simulink model "SILS_201704211"  (R2022b)
settings: Solver=ode4  StartTime=0.0  StopTime=10000  FixedStep=sim_dt  RelTol=1e-3  EnableMultiTasking=on
PreLoadFcn:
  | start
  | make_SILS
  | param_SW
  | param_sys
  | param_component
  | param_env
  | param_alignment
  | OEread
  | initialCondition
undefined symbols (not defined in the file or in its folder): ADSW, AOBC_dt, area, GAS_b2c, GGSW, GPperturbationSW, GYRO_b2c, MTQ_c2b, noise_sampling_rate, NSAS1_b2c, NSAS2_b2c, NSAS3_b2c, NSAS4_b2c, NSAS5_b2c, NSAS6_b2c, rem_mag, rem_magSW, RW_J, SRPSW, STT1_b2c_quat, STT_seed1, STT_x_noise, STT_y_noise, STT_z_noise
libraries: lib_util x23, lib_component x14, lib_env x9, aerolibutil x4, lib_orbittrance x3, aerolibtransform2 x1, sharedtransform x1
CloseFcn:
  | clean
settings Model: Creator=yamaurashusaku  LastModifiedBy=hapham
settings SolverCC: AlgebraicLoopSolver=TrustRegion
settings DataIOCC: LimitDataPoints=on  SaveFinalState=on  SaveFormat=Array  SignalLoggingSaveFormat=ModelDataLogs  SaveState=on  ReturnWorkspaceOutputs=off  StateSaveName=tmp_raccel_xout
settings OptimizationCC: ExpressionDepthLimit=2147483647  EfficientMapNaN2IntZero=off  LifeSpan=inf
settings DebuggingCC: UnderspecifiedInitializationDetection=Classic  MergeDetectMultiDrivingBlocksExec=none  SolverPrmCheckMsg=warning  MultiTaskCondExecSysMsg=warning  FcnCallInpInsideContextMsg=warning  UnconnectedInputMsg=warning  UnconnectedOutputMsg=warning  UnconnectedLineMsg=warning  StateNameClashWarn=warning  SFUnexpectedBacktrackingDiag=warning  SFNoUnconditionalDefaultTransitionDiag=warning  SFExecutionAtInitializationDiag=none  SFMachineParentedDataDiag=warning  ArithmeticOperatorsInVariantConditions=warning
settings HardwareCC: ProdBitPerPointer=32  ProdBitPerSizeT=32  ProdBitPerPtrDiffT=32  ProdLargestAtomicFloat=None  ProdIntDivRoundTo=Undefined  ProdEndianess=Unspecified  ProdWordSize=32  ProdHWDeviceType=32-bit Generic  TargetBitPerPointer=64  TargetBitPerSizeT=64  TargetBitPerPtrDiffT=64  TargetLongLongMode=on  TargetIntDivRoundTo=Zero  TargetEndianess=LittleEndian  TargetWordSize=64  TargetHWDeviceType=MATLAB Host  ProdEqTarget=off
settings ModelReferenceCC: EnableRefExpFcnMdlSchedulingChecks=on  PropagateSignalLabelsOutOfModel=off
settings SFSimCC: SimUseLocalCustomCode=off  CustomCodeUndefinedFunction=UseInterfaceOnly
settings SFSimCC: SimUserSources=|
  | sfunc_nrlmsise00_wrapper.c
  | nrlmsise-00.c
  | nrlmsise-00_data.c
  | createHandle.c
  | globals.c
  | AOCS_Process.c
settings RTWCC: SystemTargetFile=raccel.tlc  RTWVerbose=off  RTWUseLocalCustomCode=off  RTWUseSimCustomCode=on  DLArmComputeVersion=19.05
settings RTWCC: CustomSource=|
  | sfunc_nrlmsise00_wrapper.c
  | nrlmsise-00.c
  | nrlmsise-00_data.c
  | createHandle.c
  | globals.c
  | AOCS_Process.c
settings CodeAppCC: GenerateComments=off  MaxIdLength=128  SimulinkBlockComments=off
settings RaccelTargetCC: ParMdlRefBuildCompliant=off  LogVarNameModifier=rt_  OptimizeReductions=off  ENABLE_SLEXEC_SSBRIDGE=0  RTWCAPISignals=off  RTWCAPIParams=off  RTWCAPIRootIO=off
settings ConfigComp: CovMetricSettings=dw  CovSaveCumulativeToWorkspaceVar=on  CovSaveSingleToWorkspaceVar=on  CovExternalEMLEnable=off

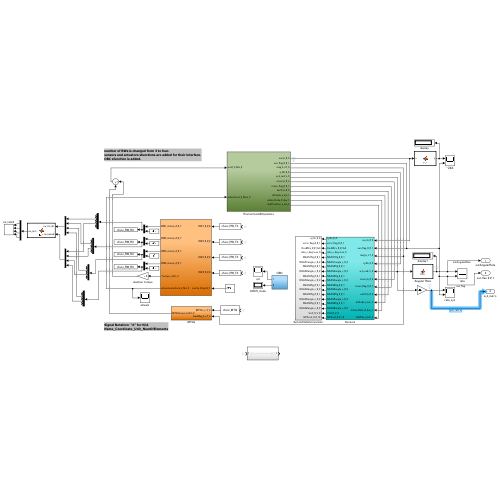
[thumbnail: Simulink's stored preview of the top-level diagram]
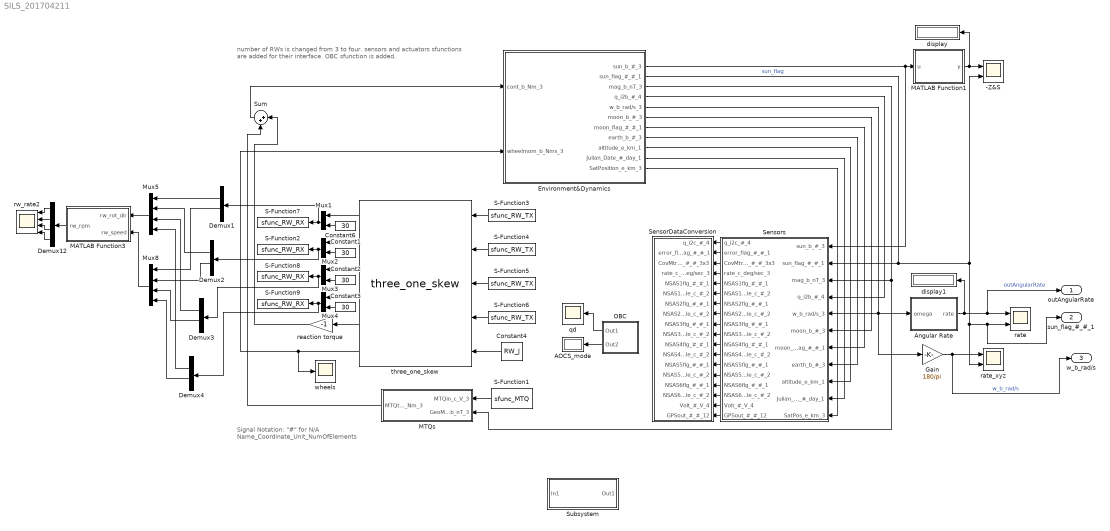
== system SILS_201704211 ==
  note: Signal Notation: "#" for N/A
      | Name_Coordinate_Unit_NumOfElements
  note: number of RWs is changed from 3 to four.
      | sensors and actuators sfunctions are added for their interface.
      | OBC sfunction is added.
  -Z&S : Scope  NumInputPorts=2
  AOCS_mode : Display
  Angular Rate : MATLAB Function  TreatAsAtomicUnit=on
  Constant{1..3,6} (4 alike) : Constant  Value=30
  Constant4 : Constant  Value=RW_J
  Demux{1..4} (4 alike) : Demux  Outputs=8
  Demux12 : Demux
  Environment&Dynamics : Subsystem
  Gain : Gain  Gain=180/pi
  MATLAB Function1 : MATLAB Function  TreatAsAtomicUnit=on
  MATLAB Function3 : MATLAB Function  TreatAsAtomicUnit=on
  MTQs : Subsystem
  Mux{1..4} (4 alike) : Mux  Inputs=2
  Mux5 : Mux
  Mux8 : Mux
  OBC : Subsystem
  S-Function1 : S-Function  FunctionName=sfunc_MTQ  Parameters=0  SFunctionDeploymentMode=off  EnableBusSupport=off
  S-Function2 : S-Function  FunctionName=sfunc_RW_RX  Parameters=1  SFunctionDeploymentMode=off  EnableBusSupport=off
  S-Function3 : S-Function  FunctionName=sfunc_RW_TX  Parameters=0  SFunctionDeploymentMode=off  EnableBusSupport=off
  S-Function4 : S-Function  FunctionName=sfunc_RW_TX  Parameters=1  SFunctionDeploymentMode=off  EnableBusSupport=off
  S-Function5 : S-Function  FunctionName=sfunc_RW_TX  Parameters=2  SFunctionDeploymentMode=off  EnableBusSupport=off
  S-Function6 : S-Function  FunctionName=sfunc_RW_TX  Parameters=3  SFunctionDeploymentMode=off  EnableBusSupport=off
  S-Function7 : S-Function  FunctionName=sfunc_RW_RX  Parameters=0  SFunctionDeploymentMode=off  EnableBusSupport=off
  S-Function8 : S-Function  FunctionName=sfunc_RW_RX  Parameters=2  SFunctionDeploymentMode=off  EnableBusSupport=off
  S-Function9 : S-Function  FunctionName=sfunc_RW_RX  Parameters=3  SFunctionDeploymentMode=off  EnableBusSupport=off
  SensorDataConversion : Subsystem
  Sensors : Subsystem
  Subsystem : Subsystem
  Sum : Sum  Inputs=|++
  display : Display
  display1 : Display
  qd : Scope
  rate : Scope  NumInputPorts=2
  rate_xyz : Scope  NumInputPorts=2
  reaction torque : Gain  Gain=-1
  rw_rate2 : Scope  NumInputPorts=4
  three_one_skew : lib_component/three_one_skew  SystemSampleTime=-1  VariantActivationTime=update diagram  Latency=0  AutoFrameSizeCalculation=off
  wheels : Scope
  outAngularRate : Outport
  sun_flag_#_#_1 : Outport  Port=2
  w_b_rad/s : Outport  Port=3
  wires:
  three_one_skew/6 -> Environment&Dynamics/2(wheelmom_b_Nms_3), wheels/1
  Environment&Dynamics/1(sun_b_#_3) -> Sensors/1(sun_b_#_3), MATLAB Function1/1(u)
  Environment&Dynamics/2(sun_flag_#_#_1) -> -Z&S/2, sun_flag_#_#_1/1, rate/2, rate_xyz/2, Sensors/2(sun_flag_#_#_1)  "sun_flag"
  Environment&Dynamics/3(mag_b_nT_3) -> Sensors/3(mag_b_nT_3), MTQs/2(GeoMag_b_nT_3)
  Environment&Dynamics/4(q_i2b_#_4) -> Sensors/4(q_i2b_#_4)
  Environment&Dynamics/5(w_b_rad/s_3) -> Angular Rate/1(omega), Sensors/5(w_b_rad/s_3), Gain/1
  Environment&Dynamics/6(moon_b_#_3) -> Sensors/6(moon_b_#_3)
  Environment&Dynamics/7(moon_flag_#_#_1) -> Sensors/7(moon_flag_#_#_1)
  Environment&Dynamics/8(earth_b_#_3) -> Sensors/8(earth_b_#_3)
  Environment&Dynamics/9(altitude_e_km_1) -> Sensors/9(altitude_e_km_1)
  Environment&Dynamics/10(Julian_Date_#_day_1) -> Sensors/10(Julian_Date_#_day_1)
  Environment&Dynamics/11(SatPosition_e_km_3) -> Sensors/11(SatPos_e_km_3)
  three_one_skew/5 -> reaction torque/1
  MTQs/1(MTQtorque_b_Nm_3) -> Sum/2
  Sum/1 -> Environment&Dynamics/1(cont_b_Nm_3)
  OBC/1(Out1) -> qd/1
  S-Function1/1 -> MTQs/1(MTQin_c_V_3)
  S-Function3/1 -> three_one_skew/1
  S-Function4/1 -> three_one_skew/2
  S-Function5/1 -> three_one_skew/3
  S-Function6/1 -> three_one_skew/4
  Mux1/1 -> Demux1/1, S-Function7/1
  three_one_skew/1 -> Mux1/1
  Constant6/1 -> Mux1/2
  Mux2/1 -> Demux2/1, S-Function2/1
  three_one_skew/2 -> Mux2/1
  Constant1/1 -> Mux2/2
  Mux3/1 -> Demux3/1, S-Function8/1
  three_one_skew/3 -> Mux3/1
  Constant2/1 -> Mux3/2
  Mux4/1 -> Demux4/1, S-Function9/1
  three_one_skew/4 -> Mux4/1
  Constant3/1 -> Mux4/2
  Constant4/1 -> three_one_skew/5
  reaction torque/1 -> Sum/1
  Gain/1 -> w_b_rad/s/1, rate_xyz/1  "w_b_rad/s"
  OBC/2(Out2) -> AOCS_mode/1
  Sensors/1(q_i2c_#_4) -> SensorDataConversion/1(q_i2c_#_4)
  Sensors/2(error_flag_#_#_1) -> SensorDataConversion/2(error_flag_#_#_1)
  Sensors/3(CovMtrx_#_#_3x3) -> SensorDataConversion/3(CovMtrx_#_#_3x3)
  Sensors/4(rate_c_deg/sec_3) -> SensorDataConversion/4(rate_c_deg/sec_3)
  Sensors/5(NSAS1flg_#_#_1) -> SensorDataConversion/5(NSAS1flg_#_#_1)
  Sensors/6(NSAS1angle_c_#_2) -> SensorDataConversion/6(NSAS1angle_c_#_2)
  Sensors/7(NSAS2flg_#_#_1) -> SensorDataConversion/7(NSAS2flg_#_#_1)
  Sensors/8(NSAS2angle_c_#_2) -> SensorDataConversion/8(NSAS2angle_c_#_2)
  Sensors/9(NSAS3flg_#_#_1) -> SensorDataConversion/9(NSAS3flg_#_#_1)
  Sensors/10(NSAS3angle_c_#_2) -> SensorDataConversion/10(NSAS3angle_c_#_2)
  Sensors/11(NSAS4flg_#_#_1) -> SensorDataConversion/11(NSAS4flg_#_#_1)
  Sensors/12(NSAS4angle_c_#_2) -> SensorDataConversion/12(NSAS4angle_c_#_2)
  Sensors/13(NSAS5flg_#_#_1) -> SensorDataConversion/13(NSAS5flg_#_#_1)
  Sensors/14(NSAS5angle_c_#_2) -> SensorDataConversion/14(NSAS5angle_c_#_2)
  Sensors/15(NSAS6flg_#_#_1) -> SensorDataConversion/15(NSAS6flg_#_#_1)
  Sensors/16(NSAS6angle_c_#_2) -> SensorDataConversion/16(NSAS6angle_c_#_2)
  Sensors/17(Volt_#_V_4) -> SensorDataConversion/17(Volt_#_V_4)
  Sensors/18(GPSout_#_#_12) -> SensorDataConversion/18(GPSout_#_#_12)
  Angular Rate/1(rate) -> display1/1, outAngularRate/1, rate/1  "outAngularRate"
  Demux1/3 -> Mux5/1
  Demux3/3 -> Mux5/3
  Demux4/3 -> Mux5/4
  Demux1/6 -> Mux8/1
  Demux2/6 -> Mux8/2
  Demux3/6 -> Mux8/3
  Demux4/6 -> Mux8/4
  MATLAB Function3/1(rw_rpm) -> Demux12/1
  Demux12/1 -> rw_rate2/1
  Demux12/2 -> rw_rate2/2
  Demux12/3 -> rw_rate2/3
  Demux12/4 -> rw_rate2/4
  Mux5/1 -> MATLAB Function3/1(rw_rot_dir)
  Mux8/1 -> MATLAB Function3/2(rw_speed)
  Demux2/3 -> Mux5/2
  MATLAB Function1/1(y) -> display/1, -Z&S/1

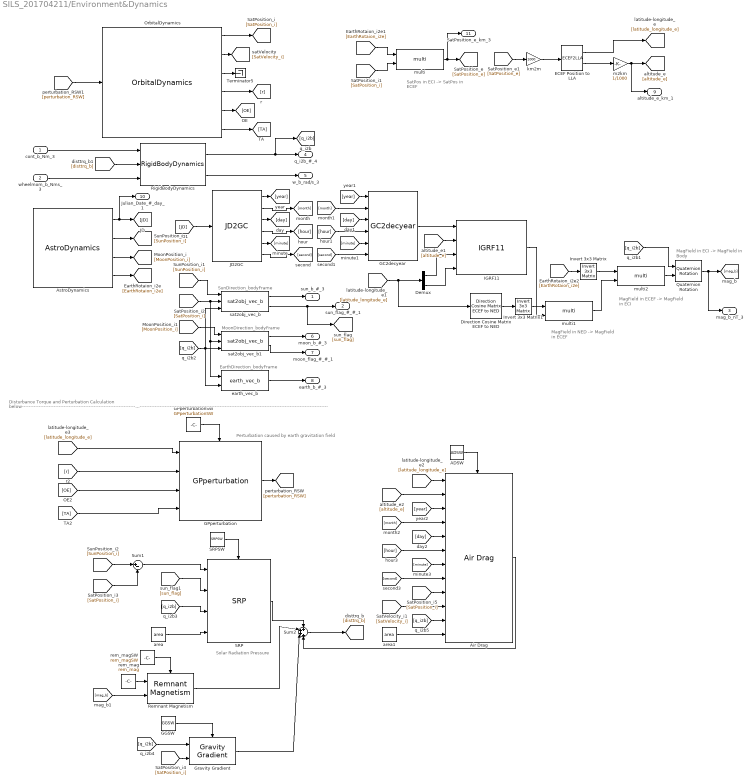
== system SILS_201704211/Environment&Dynamics ==
  note: MagField in ECI ->
      | MagField in Body
  note: MagField in ECEF ->
      | MagField in ECI
  note: MagField in NED ->
      | MagField in ECEF
  note: SatPos in ECI ->
      | SatPos in ECEF
  note: EarthDirection_bodyFrame
  note: MoonDirection_bodyFrame
  note: SunDirection_bodyFrame
  note: Disturbance Torque and Perturbation Calculation below-------------------------------------------------------------------------------------------------------------------------------------------------------------------------------------------------------------------------------------------------------------------------------------------------------------------------------------------------------
  note: Perturbation caused by earth gravitation field
  note: Solar Radiation Pressure
  cont_b_Nm_3 : Inport
  wheelmom_b_Nms_3 : Inport  Port=2
  ADSW : Constant  Value=ADSW
  Air Drag : lib_env/Environment&Dynamics/Air Drag  SystemSampleTime=-1  VariantActivationTime=update diagram  Latency=0  AutoFrameSizeCalculation=off
  AstroDynamics : lib_env/Environment&Dynamics/AstroDynamics  SystemSampleTime=-1  VariantActivationTime=update diagram  Latency=0  AutoFrameSizeCalculation=off
  Demux : Demux  Outputs=2
  Direction Cosine Matrix ECEF to NED : aerolibtransform2/Direction Cosine Matrix ECEF to NED
  ECEF Position to LLA : ECEF2LLA  R=6378137
  GC2decyear : lib_util/GC2decyear  SystemSampleTime=-1  VariantActivationTime=update diagram  Latency=0  AutoFrameSizeCalculation=off
  GGSW : Constant  Value=GGSW
  GPperturbation : lib_env/Environment&Dynamics/GPperturbation  SystemSampleTime=-1  VariantActivationTime=update diagram  Latency=0  AutoFrameSizeCalculation=off
  GPperturbationSW : Constant  Value=GPperturbationSW
  Gravity Gradient : lib_env/Environment&Dynamics/Gravity Gradient  SystemSampleTime=-1  VariantActivationTime=update diagram  Latency=0  AutoFrameSizeCalculation=off
  IGRF11 : lib_env/IGRF11  SystemSampleTime=-1  VariantActivationTime=update diagram  Latency=0  AutoFrameSizeCalculation=off
  Invert 3x3 Matrix : aerolibutil/Invert  3x3 Matrix
  Invert 3x3 Matrix1 : aerolibutil/Invert  3x3 Matrix
  JD2GC : lib_util/JD2GC  SystemSampleTime=-1  VariantActivationTime=update diagram  Latency=0  AutoFrameSizeCalculation=off
  OrbitalDynamics : lib_env/Environment&Dynamics/OrbitalDynamics  SystemSampleTime=-1  VariantActivationTime=update diagram  Latency=0  AutoFrameSizeCalculation=off
  Quaternion Rotation : aerolibutil/Quaternion Rotation
  Remnant Magnetism : lib_env/Environment&Dynamics/Remnant Magnetism  SystemSampleTime=-1  VariantActivationTime=update diagram  Latency=0  AutoFrameSizeCalculation=off
  RigidBodyDynamics : lib_env/Environment&Dynamics/RigidBodyDynamics  SystemSampleTime=-1  VariantActivationTime=update diagram  Latency=0  AutoFrameSizeCalculation=off
  SRP : lib_env/Environment&Dynamics/SRP  SystemSampleTime=-1  VariantActivationTime=update diagram  Latency=0  AutoFrameSizeCalculation=off
  SRPSW : Constant  Value=SRPSW
  Sum1 : Sum  Inputs=|+-
  Sum2 : Sum  Inputs=++++
  Terminator5 : Terminator
  area : Constant  Value=area
  area1 : Constant  Value=area
  earth_vec_b : lib_orbittrance/earth_vec_b  SystemSampleTime=-1  VariantActivationTime=update diagram  Latency=0  AutoFrameSizeCalculation=off
  km2m : Gain  Gain=1000
  m2km : Gain  Gain=1/1000
  multi : lib_util/multi  SystemSampleTime=-1  VariantActivationTime=update diagram  Latency=0  AutoFrameSizeCalculation=off
  multi1 : lib_util/multi  SystemSampleTime=-1  VariantActivationTime=update diagram  Latency=0  AutoFrameSizeCalculation=off
  multi2 : lib_util/multi  SystemSampleTime=-1  VariantActivationTime=update diagram  Latency=0  AutoFrameSizeCalculation=off
  rem_mag : Constant  Value=rem_mag
  rem_magSW : Constant  Value=rem_magSW
  sat2obj_vec_b : lib_orbittrance/sat2obj_vec_b  SystemSampleTime=-1  VariantActivationTime=update diagram  Latency=0  AutoFrameSizeCalculation=off
  sat2obj_vec_b1 : lib_orbittrance/sat2obj_vec_b  SystemSampleTime=-1  VariantActivationTime=update diagram  Latency=0  AutoFrameSizeCalculation=off
  sun_b_#_3 : Outport
  sun_flag_#_#_1 : Outport  Port=2
  mag_b_nT_3 : Outport  Port=3
  q_i2b_#_4 : Outport  Port=4
  w_b_rad/s_3 : Outport  Port=5
  moon_b_#_3 : Outport  Port=6
  moon_flag_#_#_1 : Outport  Port=7
  earth_b_#_3 : Outport  Port=8
  altitude_e_km_1 : Outport  Port=9
  Julian_Date_#_day_1 : Outport  Port=10
  SatPosition_e_km_3 : Outport  Port=11
  wires:
  RigidBodyDynamics/1 -> q_i2b_#_4/1, [q_i2b]
  RigidBodyDynamics/2 -> w_b_rad/s_3/1
  cont_b_Nm_3/1 -> RigidBodyDynamics/1
  wheelmom_b_Nms_3/1 -> RigidBodyDynamics/3
  AstroDynamics/1 -> [JD], Julian_Date_#_day_1/1
  AstroDynamics/4 -> [EarthRotaion_i2e]
  [second] -> GC2decyear/6
  [minute] -> GC2decyear/5
  [hour] -> GC2decyear/4
  [day] -> GC2decyear/3
  [month] -> GC2decyear/2
  [year] -> GC2decyear/1
  JD2GC/6 -> [second]
  JD2GC/5 -> [minute]
  JD2GC/4 -> [hour]
  JD2GC/3 -> [day]
  JD2GC/2 -> [month]
  JD2GC/1 -> [year]
  Quaternion Rotation/1 -> mag_b_nT_3/1, [mag_b]
  [q_i2b] -> Quaternion Rotation/1
  multi2/1 -> Quaternion Rotation/2
  multi1/1 -> multi2/2
  Invert 3x3 Matrix/1 -> multi2/1
  [EarthRotaion_i2e] -> Invert 3x3 Matrix/1
  IGRF11/1 -> multi1/2
  Invert 3x3 Matrix1/1 -> multi1/1
  Direction Cosine Matrix ECEF to NED/1 -> Invert 3x3 Matrix1/1
  Demux/2 -> IGRF11/4
  Demux/1 -> IGRF11/3
  [altitude_e] -> IGRF11/2
  [latitude_longitude_e] -> Direction Cosine Matrix ECEF to NED/1, Demux/1
  [JD] -> JD2GC/1
  GC2decyear/1 -> IGRF11/1
  ECEF Position to LLA/1 -> [latitude_longitude_e]
  m2km/1 -> [altitude_e], altitude_e_km_1/1
  ECEF Position to LLA/2 -> m2km/1
  km2m/1 -> ECEF Position to LLA/1
  [SatPosition_e] -> km2m/1
  multi/1 -> [SatPosition_e], SatPosition_e_km_3/1
  [SatPosition_i] -> multi/2
  [EarthRotaion_i2e] -> multi/1
  OrbitalDynamics/1 -> [SatPosition_i]
  OrbitalDynamics/2 -> [SatVelocity_i]
  OrbitalDynamics/4 -> [r]
  OrbitalDynamics/5 -> [OE]
  OrbitalDynamics/6 -> [TA]
  AstroDynamics/2 -> [SunPosition_i]
  AstroDynamics/3 -> [MoonPosition_i]
  earth_vec_b/1 -> earth_b_#_3/1
  sat2obj_vec_b1/2 -> moon_flag_#_#_1/1
  sat2obj_vec_b1/1 -> moon_b_#_3/1
  sat2obj_vec_b/1 -> sun_b_#_3/1
  sat2obj_vec_b/2 -> sun_flag_#_#_1/1, [sun_flag]
  [SunPosition_i] -> sat2obj_vec_b/1
  [MoonPosition_i] -> sat2obj_vec_b1/1
  [q_i2b] -> sat2obj_vec_b/3, earth_vec_b/2, sat2obj_vec_b1/3
  [SatPosition_i] -> sat2obj_vec_b/2, sat2obj_vec_b1/2, earth_vec_b/1
  OrbitalDynamics/3 -> Terminator5/1
  GPperturbation/1 -> [perturbation_RSW]
  Gravity Gradient/1 -> Sum2/3
  Remnant Magnetism/1 -> Sum2/2
  [latitude_longitude_e] -> GPperturbation/1
  [r] -> GPperturbation/2
  [OE] -> GPperturbation/3
  [TA] -> GPperturbation/4
  GPperturbationSW/1 -> GPperturbation/Enable
  Sum1/1 -> SRP/1
  [sun_flag] -> SRP/2
  area/1 -> SRP/4
  [q_i2b] -> SRP/3
  [SatPosition_i] -> Sum1/2
  [SunPosition_i] -> Sum1/1
  SRPSW/1 -> SRP/Enable
  rem_mag/1 -> Remnant Magnetism/1
  [mag_b] -> Remnant Magnetism/2
  rem_magSW/1 -> Remnant Magnetism/Enable
  Sum2/1 -> [disttrq_b]
  SRP/1 -> Sum2/1
  [q_i2b] -> Gravity Gradient/1
  [SatPosition_i] -> Gravity Gradient/2
  GGSW/1 -> Gravity Gradient/Enable
  [latitude_longitude_e] -> Air Drag/1
  [altitude_e] -> Air Drag/2
  [month] -> Air Drag/4
  [day] -> Air Drag/5
  [hour] -> Air Drag/6
  [minute] -> Air Drag/7
  [second] -> Air Drag/8
  [SatPosition_i] -> Air Drag/9
  [SatVelocity_i] -> Air Drag/10
  area1/1 -> Air Drag/12
  [q_i2b] -> Air Drag/11
  [year] -> Air Drag/3
  ADSW/1 -> Air Drag/Enable
  Air Drag/1 -> Sum2/4
  [disttrq_b] -> RigidBodyDynamics/2
  [perturbation_RSW] -> OrbitalDynamics/1

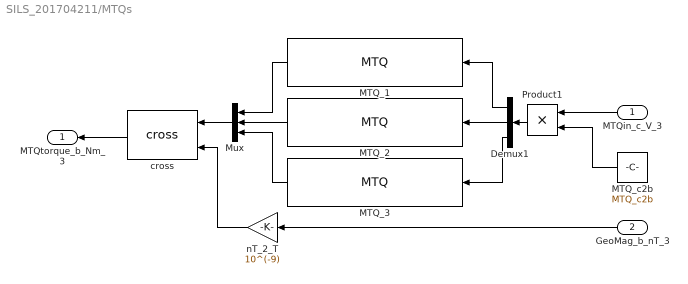
== system SILS_201704211/MTQs ==
  MTQin_c_V_3 : Inport
  GeoMag_b_nT_3 : Inport  Port=2
  Demux1 : Demux  Outputs=3
  MTQ_1 : lib_component/MTQ  SystemSampleTime=-1  VariantActivationTime=update diagram  Latency=0  AutoFrameSizeCalculation=off
  MTQ_2 : lib_component/MTQ  SystemSampleTime=-1  VariantActivationTime=update diagram  Latency=0  AutoFrameSizeCalculation=off
  MTQ_3 : lib_component/MTQ  SystemSampleTime=-1  VariantActivationTime=update diagram  Latency=0  AutoFrameSizeCalculation=off
  MTQ_c2b : Constant  Value=MTQ_c2b
  Mux : Mux  Inputs=3
  Product1 : Product  RndMeth=Zero
  cross : lib_util/cross  SystemSampleTime=-1  VariantActivationTime=update diagram  Latency=0  AutoFrameSizeCalculation=off
  nT_2_T : Gain  Gain=10^(-9)
  MTQtorque_b_Nm_3 : Outport
  wires:
  MTQ_1/1 -> Mux/1
  MTQ_2/1 -> Mux/2
  MTQ_3/1 -> Mux/3
  Mux/1 -> cross/1
  Demux1/1 -> MTQ_1/1
  Demux1/2 -> MTQ_2/1
  Demux1/3 -> MTQ_3/1
  nT_2_T/1 -> cross/2
  GeoMag_b_nT_3/1 -> nT_2_T/1
  MTQ_c2b/1 -> Product1/2
  Product1/1 -> Demux1/1
  MTQin_c_V_3/1 -> Product1/1
  cross/1 -> MTQtorque_b_Nm_3/1

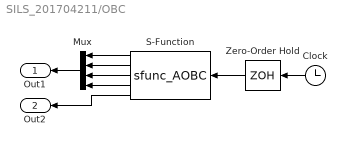
== system SILS_201704211/OBC ==
  Clock : Clock
  Mux : Mux
  S-Function : S-Function  FunctionName=sfunc_AOBC  SFunctionDeploymentMode=off  EnableBusSupport=off
  Zero-Order Hold : ZeroOrderHold  SampleTime=AOBC_dt
  Out1 : Outport
  Out2 : Outport  Port=2
  wires:
  Clock/1 -> Zero-Order Hold/1
  Zero-Order Hold/1 -> S-Function/1
  S-Function/1 -> Mux/1
  S-Function/2 -> Mux/2
  S-Function/3 -> Mux/3
  S-Function/4 -> Mux/4
  Mux/1 -> Out1/1
  S-Function/5 -> Out2/1

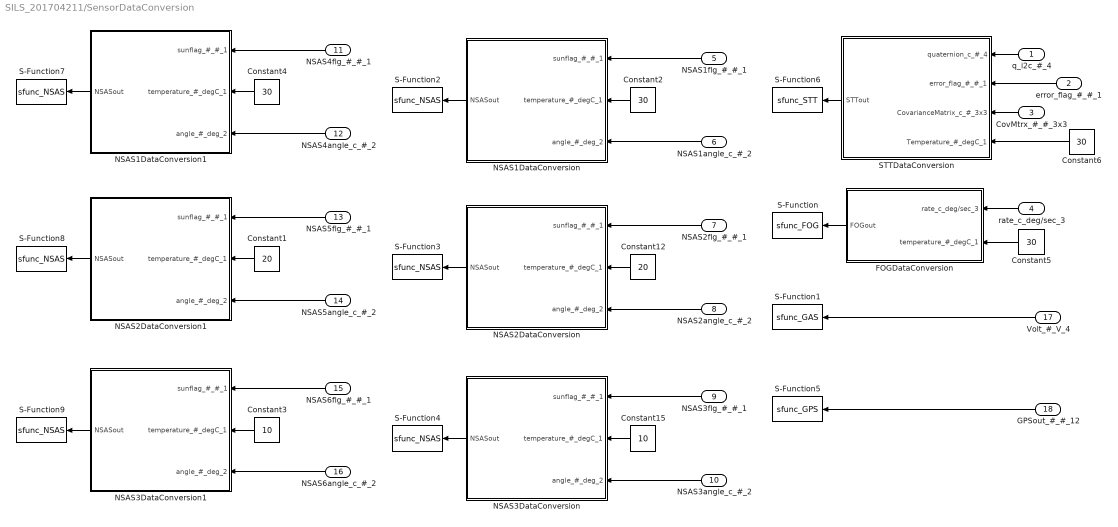
== system SILS_201704211/SensorDataConversion ==
  q_i2c_#_4 : Inport
  error_flag_#_#_1 : Inport  Port=2
  CovMtrx_#_#_3x3 : Inport  Port=3
  rate_c_deg/sec_3 : Inport  Port=4
  NSAS1flg_#_#_1 : Inport  Port=5
  NSAS1angle_c_#_2 : Inport  Port=6
  NSAS2flg_#_#_1 : Inport  Port=7
  NSAS2angle_c_#_2 : Inport  Port=8
  NSAS3flg_#_#_1 : Inport  Port=9
  NSAS3angle_c_#_2 : Inport  Port=10
  NSAS4flg_#_#_1 : Inport  Port=11
  NSAS4angle_c_#_2 : Inport  Port=12
  NSAS5flg_#_#_1 : Inport  Port=13
  NSAS5angle_c_#_2 : Inport  Port=14
  NSAS6flg_#_#_1 : Inport  Port=15
  NSAS6angle_c_#_2 : Inport  Port=16
  Volt_#_V_4 : Inport  Port=17
  GPSout_#_#_12 : Inport  Port=18
  Constant1 : Constant  Value=20
  Constant12 : Constant  Value=20
  Constant15 : Constant  Value=10
  Constant2 : Constant  Value=30
  Constant3 : Constant  Value=10
  Constant4 : Constant  Value=30
  Constant5 : Constant  Value=30  SampleTime=0
  Constant6 : Constant  Value=30
  FOGDataConversion : Subsystem
  NSAS1DataConversion : Subsystem
  NSAS1DataConversion1 : Subsystem
  NSAS2DataConversion : Subsystem
  NSAS2DataConversion1 : Subsystem
  NSAS3DataConversion : Subsystem
  NSAS3DataConversion1 : Subsystem
  S-Function : S-Function  FunctionName=sfunc_FOG  Parameters=0 2  SFunctionDeploymentMode=off  EnableBusSupport=off
  S-Function1 : S-Function  FunctionName=sfunc_GAS  Parameters=0  SFunctionDeploymentMode=off  EnableBusSupport=off
  S-Function2 : S-Function  FunctionName=sfunc_NSAS  Parameters=0 0  SFunctionDeploymentMode=off  EnableBusSupport=off
  S-Function3 : S-Function  FunctionName=sfunc_NSAS  Parameters=1 1  SFunctionDeploymentMode=off  EnableBusSupport=off
  S-Function4 : S-Function  FunctionName=sfunc_NSAS  Parameters=2 2  SFunctionDeploymentMode=off  EnableBusSupport=off
  S-Function5 : S-Function  FunctionName=sfunc_GPS  Parameters=0  SFunctionDeploymentMode=off  EnableBusSupport=off
  S-Function6 : S-Function  FunctionName=sfunc_STT  Parameters=0 1  SFunctionDeploymentMode=off  EnableBusSupport=off
  S-Function7 : S-Function  FunctionName=sfunc_NSAS  Parameters=3 3  SFunctionDeploymentMode=off  EnableBusSupport=off
  S-Function8 : S-Function  FunctionName=sfunc_NSAS  Parameters=4 4  SFunctionDeploymentMode=off  EnableBusSupport=off
  S-Function9 : S-Function  FunctionName=sfunc_NSAS  Parameters=5 5  SFunctionDeploymentMode=off  EnableBusSupport=off
  STTDataConversion : Subsystem
  wires:
  Constant5/1 -> FOGDataConversion/2(temperature_#_degC_1)
  Constant2/1 -> NSAS1DataConversion/2(temperature_#_degC_1)
  NSAS1flg_#_#_1/1 -> NSAS1DataConversion/1(sunflag_#_#_1)
  NSAS1angle_c_#_2/1 -> NSAS1DataConversion/3(angle_#_deg_2)
  NSAS2flg_#_#_1/1 -> NSAS2DataConversion/1(sunflag_#_#_1)
  NSAS2angle_c_#_2/1 -> NSAS2DataConversion/3(angle_#_deg_2)
  Constant12/1 -> NSAS2DataConversion/2(temperature_#_degC_1)
  Constant15/1 -> NSAS3DataConversion/2(temperature_#_degC_1)
  NSAS3flg_#_#_1/1 -> NSAS3DataConversion/1(sunflag_#_#_1)
  NSAS3angle_c_#_2/1 -> NSAS3DataConversion/3(angle_#_deg_2)
  q_i2c_#_4/1 -> STTDataConversion/1(quaternion_c_#_4)
  error_flag_#_#_1/1 -> STTDataConversion/2(error_flag_#_#_1)
  CovMtrx_#_#_3x3/1 -> STTDataConversion/3(CovarianceMatrix_c_#_3x3)
  Constant6/1 -> STTDataConversion/4(Temperature_#_degC_1)
  rate_c_deg/sec_3/1 -> FOGDataConversion/1(rate_c_deg/sec_3)
  NSAS3DataConversion/1(NSASout) -> S-Function4/1
  NSAS2DataConversion/1(NSASout) -> S-Function3/1
  NSAS1DataConversion/1(NSASout) -> S-Function2/1
  GPSout_#_#_12/1 -> S-Function5/1
  Volt_#_V_4/1 -> S-Function1/1
  FOGDataConversion/1(FOGout) -> S-Function/1
  STTDataConversion/1(STTout) -> S-Function6/1
  Constant4/1 -> NSAS1DataConversion1/2(temperature_#_degC_1)
  NSAS4flg_#_#_1/1 -> NSAS1DataConversion1/1(sunflag_#_#_1)
  NSAS4angle_c_#_2/1 -> NSAS1DataConversion1/3(angle_#_deg_2)
  NSAS5flg_#_#_1/1 -> NSAS2DataConversion1/1(sunflag_#_#_1)
  NSAS5angle_c_#_2/1 -> NSAS2DataConversion1/3(angle_#_deg_2)
  Constant1/1 -> NSAS2DataConversion1/2(temperature_#_degC_1)
  Constant3/1 -> NSAS3DataConversion1/2(temperature_#_degC_1)
  NSAS6flg_#_#_1/1 -> NSAS3DataConversion1/1(sunflag_#_#_1)
  NSAS6angle_c_#_2/1 -> NSAS3DataConversion1/3(angle_#_deg_2)
  NSAS3DataConversion1/1(NSASout) -> S-Function9/1
  NSAS2DataConversion1/1(NSASout) -> S-Function8/1
  NSAS1DataConversion1/1(NSASout) -> S-Function7/1

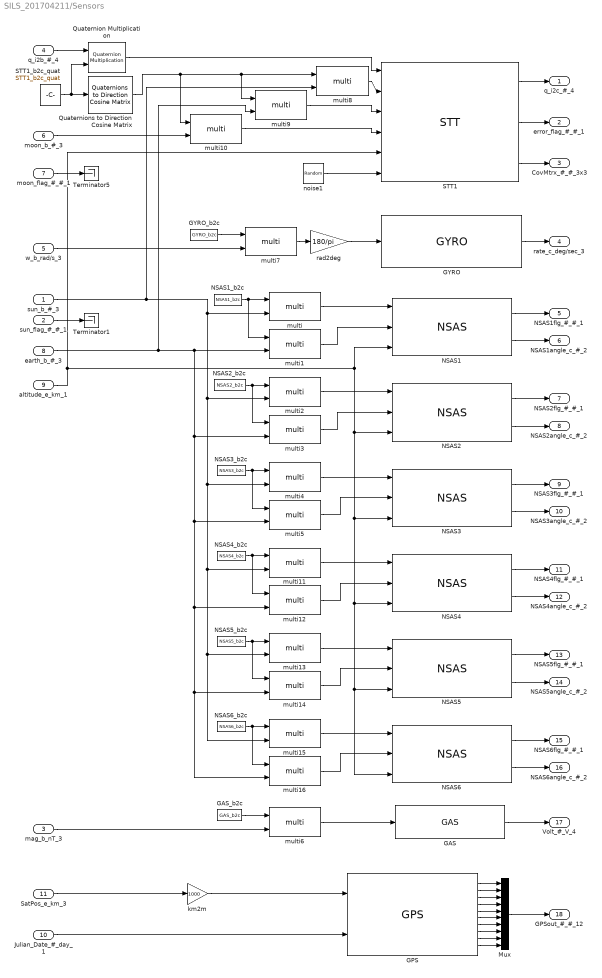
== system SILS_201704211/Sensors ==
  sun_b_#_3 : Inport
  sun_flag_#_#_1 : Inport  Port=2
  mag_b_nT_3 : Inport  Port=3
  q_i2b_#_4 : Inport  Port=4
  w_b_rad/s_3 : Inport  Port=5
  moon_b_#_3 : Inport  Port=6
  moon_flag_#_#_1 : Inport  Port=7
  earth_b_#_3 : Inport  Port=8
  altitude_e_km_1 : Inport  Port=9
  Julian_Date_#_day_1 : Inport  Port=10
  SatPos_e_km_3 : Inport  Port=11
  GAS : lib_component/GAS  SystemSampleTime=-1  VariantActivationTime=update diagram  Latency=0  AutoFrameSizeCalculation=off
  GAS_b2c : Constant  Value=GAS_b2c  VectorParams1D=off
  GPS : lib_component/GPS  SystemSampleTime=-1  VariantActivationTime=update diagram  Latency=0  AutoFrameSizeCalculation=off
  GYRO : lib_component/GYRO  SystemSampleTime=-1  VariantActivationTime=update diagram  Latency=0  AutoFrameSizeCalculation=off
  GYRO_b2c : Constant  Value=GYRO_b2c  VectorParams1D=off
  Mux : Mux  Inputs=10
  NSAS{1..6} (6 alike) : lib_component/NSAS  SystemSampleTime=-1  VariantActivationTime=update diagram  Latency=0  AutoFrameSizeCalculation=off
  NSAS1_b2c : Constant  Value=NSAS1_b2c  VectorParams1D=off
  NSAS2_b2c : Constant  Value=NSAS2_b2c  VectorParams1D=off
  NSAS3_b2c : Constant  Value=NSAS3_b2c  VectorParams1D=off
  NSAS4_b2c : Constant  Value=NSAS4_b2c  VectorParams1D=off
  NSAS5_b2c : Constant  Value=NSAS5_b2c  VectorParams1D=off
  NSAS6_b2c : Constant  Value=NSAS6_b2c  VectorParams1D=off
  Quaternion Multiplication : aerolibutil/Quaternion Multiplication
  Quaternions to Direction Cosine Matrix : sharedtransform/Quaternions to  Direction Cosine Matrix  aMode=aMode
  STT1 : lib_component/STT  SystemSampleTime=-1  VariantActivationTime=update diagram  Latency=0  AutoFrameSizeCalculation=off
  STT1_b2c_quat : Constant  Value=STT1_b2c_quat
  Terminator1 : Terminator
  Terminator5 : Terminator
  km2m : Gain  Gain=1000
  multi{,1..16} (17 alike) : lib_util/multi  SystemSampleTime=-1  VariantActivationTime=update diagram  Latency=0  AutoFrameSizeCalculation=off
  noise1 : RandomNumber  Mean=[0 0 0]  Variance=[STT_x_noise*STT_x_noise STT_y_noise*STT_y_noise STT_z_noise*STT_z_noise]  Seed=STT_seed1  SampleTime=noise_sampling_rate
  rad2deg : Gain  Gain=180/pi
  q_i2c_#_4 : Outport
  error_flag_#_#_1 : Outport  Port=2
  CovMtrx_#_#_3x3 : Outport  Port=3
  rate_c_deg/sec_3 : Outport  Port=4
  NSAS1flg_#_#_1 : Outport  Port=5
  NSAS1angle_c_#_2 : Outport  Port=6
  NSAS2flg_#_#_1 : Outport  Port=7
  NSAS2angle_c_#_2 : Outport  Port=8
  NSAS3flg_#_#_1 : Outport  Port=9
  NSAS3angle_c_#_2 : Outport  Port=10
  NSAS4flg_#_#_1 : Outport  Port=11
  NSAS4angle_c_#_2 : Outport  Port=12
  NSAS5flg_#_#_1 : Outport  Port=13
  NSAS5angle_c_#_2 : Outport  Port=14
  NSAS6flg_#_#_1 : Outport  Port=15
  NSAS6angle_c_#_2 : Outport  Port=16
  Volt_#_V_4 : Outport  Port=17
  GPSout_#_#_12 : Outport  Port=18
  wires:
  Mux/1 -> GPSout_#_#_12/1
  GAS/1 -> Volt_#_V_4/1
  NSAS3/2 -> NSAS3angle_c_#_2/1
  NSAS3/1 -> NSAS3flg_#_#_1/1
  NSAS2/2 -> NSAS2angle_c_#_2/1
  NSAS2/1 -> NSAS2flg_#_#_1/1
  NSAS1/2 -> NSAS1angle_c_#_2/1
  NSAS1/1 -> NSAS1flg_#_#_1/1
  GYRO/1 -> rate_c_deg/sec_3/1
  STT1/3 -> CovMtrx_#_#_3x3/1
  STT1/2 -> error_flag_#_#_1/1
  STT1/1 -> q_i2c_#_4/1
  moon_b_#_3/1 -> multi10/2
  GYRO_b2c/1 -> multi7/1
  w_b_rad/s_3/1 -> multi7/2
  mag_b_nT_3/1 -> multi6/2
  GAS_b2c/1 -> multi6/1
  NSAS3_b2c/1 -> multi5/1, multi4/1
  multi5/1 -> NSAS3/2
  NSAS2_b2c/1 -> multi3/1, multi2/1
  NSAS1_b2c/1 -> multi1/1, multi/1
  multi1/1 -> NSAS1/2
  multi9/1 -> STT1/3
  GPS/10 -> Mux/10
  GPS/9 -> Mux/9
  GPS/8 -> Mux/8
  GPS/7 -> Mux/7
  GPS/6 -> Mux/6
  GPS/5 -> Mux/5
  GPS/4 -> Mux/4
  GPS/3 -> Mux/3
  GPS/2 -> Mux/2
  GPS/1 -> Mux/1
  SatPos_e_km_3/1 -> km2m/1
  Julian_Date_#_day_1/1 -> GPS/2
  multi10/1 -> STT1/4
  multi8/1 -> STT1/2
  multi4/1 -> NSAS3/1
  multi3/1 -> NSAS2/2
  multi2/1 -> NSAS2/1
  multi6/1 -> GAS/1
  multi/1 -> NSAS1/1
  rad2deg/1 -> GYRO/1
  multi7/1 -> rad2deg/1
  km2m/1 -> GPS/1
  q_i2b_#_4/1 -> Quaternion Multiplication/1
  Quaternion Multiplication/1 -> STT1/1
  STT1_b2c_quat/1 -> Quaternion Multiplication/2, Quaternions to Direction Cosine Matrix/1
  Quaternions to Direction Cosine Matrix/1 -> multi10/1, multi9/1, multi8/1
  noise1/1 -> STT1/6
  moon_flag_#_#_1/1 -> Terminator5/1
  sun_flag_#_#_1/1 -> Terminator1/1
  NSAS4_b2c/1 -> multi11/1, multi12/1
  multi12/1 -> NSAS4/2
  multi11/1 -> NSAS4/1
  NSAS4/1 -> NSAS4flg_#_#_1/1
  NSAS4/2 -> NSAS4angle_c_#_2/1
  NSAS5_b2c/1 -> multi14/1, multi13/1
  multi14/1 -> NSAS5/2
  multi13/1 -> NSAS5/1
  NSAS5/1 -> NSAS5flg_#_#_1/1
  NSAS5/2 -> NSAS5angle_c_#_2/1
  NSAS6_b2c/1 -> multi16/1, multi15/1
  multi16/1 -> NSAS6/2
  multi15/1 -> NSAS6/1
  altitude_e_km_1/1 -> NSAS6/3, NSAS5/3, NSAS4/3, NSAS3/3, NSAS2/3, NSAS1/3, STT1/5
  earth_b_#_3/1 -> multi5/2, multi14/2, multi16/2, multi12/2, multi3/2, multi1/2, multi9/2
  sun_b_#_3/1 -> multi4/2, multi11/2, multi13/2, multi15/2, multi2/2, multi/2, multi8/2
  NSAS6/1 -> NSAS6flg_#_#_1/1
  NSAS6/2 -> NSAS6angle_c_#_2/1

== system SILS_201704211/Subsystem ==
  In1 : Inport
  Out1 : Outport
  wires:
  In1/1 -> Out1/1

== system SILS_201704211/SensorDataConversion/FOGDataConversion ==
  rate_c_deg/sec_3 : Inport
  temperature_#_degC_1 : Inport  Port=2
  Mux : Mux  Inputs=2
  FOGout : Outport
  wires:
  Mux/1 -> FOGout/1
  rate_c_deg/sec_3/1 -> Mux/1
  temperature_#_degC_1/1 -> Mux/2

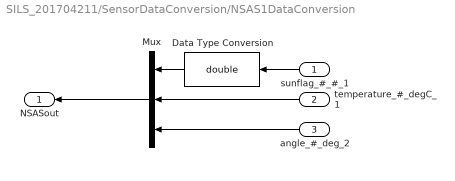
== system SILS_201704211/SensorDataConversion/NSAS1DataConversion ==
  sunflag_#_#_1 : Inport
  temperature_#_degC_1 : Inport  Port=2
  angle_#_deg_2 : Inport  Port=3
  Data Type Conversion : DataTypeConversion  OutDataTypeStr=double  SaturateOnIntegerOverflow=off  RndMeth=Floor
  Mux : Mux  Inputs=3
  NSASout : Outport
  wires:
  Mux/1 -> NSASout/1
  sunflag_#_#_1/1 -> Data Type Conversion/1
  angle_#_deg_2/1 -> Mux/3
  Data Type Conversion/1 -> Mux/1
  temperature_#_degC_1/1 -> Mux/2

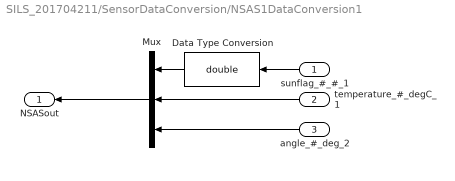
== system SILS_201704211/SensorDataConversion/NSAS1DataConversion1 ==
  sunflag_#_#_1 : Inport
  temperature_#_degC_1 : Inport  Port=2
  angle_#_deg_2 : Inport  Port=3
  Data Type Conversion : DataTypeConversion  OutDataTypeStr=double  SaturateOnIntegerOverflow=off  RndMeth=Floor
  Mux : Mux  Inputs=3
  NSASout : Outport
  wires:
  temperature_#_degC_1/1 -> Mux/2
  Data Type Conversion/1 -> Mux/1
  angle_#_deg_2/1 -> Mux/3
  sunflag_#_#_1/1 -> Data Type Conversion/1
  Mux/1 -> NSASout/1

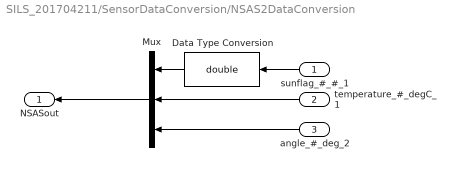
== system SILS_201704211/SensorDataConversion/NSAS2DataConversion ==
  sunflag_#_#_1 : Inport
  temperature_#_degC_1 : Inport  Port=2
  angle_#_deg_2 : Inport  Port=3
  Data Type Conversion : DataTypeConversion  OutDataTypeStr=double  SaturateOnIntegerOverflow=off  RndMeth=Floor
  Mux : Mux  Inputs=3
  NSASout : Outport
  wires:
  temperature_#_degC_1/1 -> Mux/2
  Data Type Conversion/1 -> Mux/1
  angle_#_deg_2/1 -> Mux/3
  sunflag_#_#_1/1 -> Data Type Conversion/1
  Mux/1 -> NSASout/1

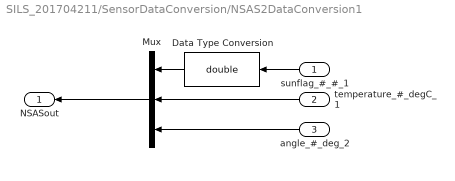
== system SILS_201704211/SensorDataConversion/NSAS2DataConversion1 ==
  sunflag_#_#_1 : Inport
  temperature_#_degC_1 : Inport  Port=2
  angle_#_deg_2 : Inport  Port=3
  Data Type Conversion : DataTypeConversion  OutDataTypeStr=double  SaturateOnIntegerOverflow=off  RndMeth=Floor
  Mux : Mux  Inputs=3
  NSASout : Outport
  wires:
  Mux/1 -> NSASout/1
  sunflag_#_#_1/1 -> Data Type Conversion/1
  angle_#_deg_2/1 -> Mux/3
  Data Type Conversion/1 -> Mux/1
  temperature_#_degC_1/1 -> Mux/2

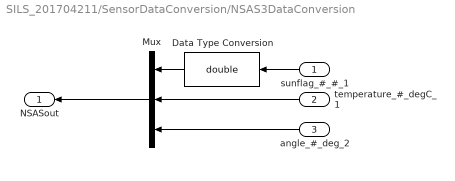
== system SILS_201704211/SensorDataConversion/NSAS3DataConversion ==
  sunflag_#_#_1 : Inport
  temperature_#_degC_1 : Inport  Port=2
  angle_#_deg_2 : Inport  Port=3
  Data Type Conversion : DataTypeConversion  OutDataTypeStr=double  SaturateOnIntegerOverflow=off  RndMeth=Floor
  Mux : Mux  Inputs=3
  NSASout : Outport
  wires:
  Mux/1 -> NSASout/1
  sunflag_#_#_1/1 -> Data Type Conversion/1
  angle_#_deg_2/1 -> Mux/3
  Data Type Conversion/1 -> Mux/1
  temperature_#_degC_1/1 -> Mux/2

== system SILS_201704211/SensorDataConversion/NSAS3DataConversion1 ==
  sunflag_#_#_1 : Inport
  temperature_#_degC_1 : Inport  Port=2
  angle_#_deg_2 : Inport  Port=3
  Data Type Conversion : DataTypeConversion  OutDataTypeStr=double  SaturateOnIntegerOverflow=off  RndMeth=Floor
  Mux : Mux  Inputs=3
  NSASout : Outport
  wires:
  temperature_#_degC_1/1 -> Mux/2
  Data Type Conversion/1 -> Mux/1
  angle_#_deg_2/1 -> Mux/3
  sunflag_#_#_1/1 -> Data Type Conversion/1
  Mux/1 -> NSASout/1

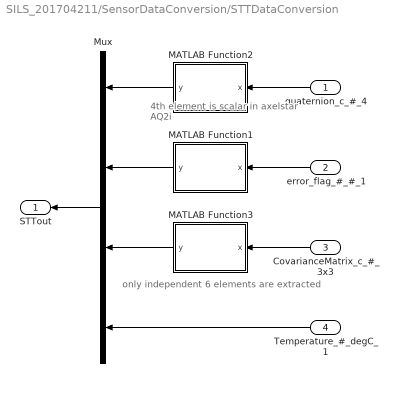
== system SILS_201704211/SensorDataConversion/STTDataConversion ==
  note: 4th element is scalar in axelstar
      | AQ2i
  note: only independent 6 elements are extracted
  quaternion_c_#_4 : Inport
  error_flag_#_#_1 : Inport  Port=2
  CovarianceMatrix_c_#_3x3 : Inport  Port=3
  Temperature_#_degC_1 : Inport  Port=4
  MATLAB Function1 : MATLAB Function  TreatAsAtomicUnit=on
  MATLAB Function2 : MATLAB Function  TreatAsAtomicUnit=on
  MATLAB Function3 : MATLAB Function  TreatAsAtomicUnit=on
  Mux : Mux
  STTout : Outport
  wires:
  quaternion_c_#_4/1 -> MATLAB Function2/1(x)
  CovarianceMatrix_c_#_3x3/1 -> MATLAB Function3/1(x)
  MATLAB Function2/1(y) -> Mux/1
  Mux/1 -> STTout/1
  error_flag_#_#_1/1 -> MATLAB Function1/1(x)
  Temperature_#_degC_1/1 -> Mux/4
  MATLAB Function1/1(y) -> Mux/2
  MATLAB Function3/1(y) -> Mux/3

== matlab function SILS_201704211/MATLAB Function3 ==
  data: rw_rot_dir input; rw_rpm output; rw_speed input
function rw_rpm = fcn(rw_rot_dir,rw_speed)
%#codegen

if rw_rot_dir(1)>0.5
    rw_speed_1 = -rw_speed(1);
else
    rw_speed_1 = rw_speed(1);
end

if rw_rot_dir(2)>0.5
    rw_speed_2 = -rw_speed(2);
else
    rw_speed_2 = rw_speed(2);
end

if rw_rot_dir(3)>0.5
    rw_speed_3 = -rw_speed(3);
else
    rw_speed_3 = rw_speed(3);
end

if rw_rot_dir(4)>0.5
    rw_speed_4 = -rw_speed(4);
else
    rw_speed_4 = rw_speed(4);
end

rw_rpm = [rw_speed_1 rw_speed_2 rw_speed_3 rw_speed_4];

== matlab function SILS_201704211/Angular Rate ==
  data: omega input; rate output
function rate = fcn(omega)
%#codegen

rate = sqrt(omega(1)^2+omega(2)^2+omega(3)^2) *180/pi;

== matlab function SILS_201704211/SensorDataConversion/STTDataConversion/MATLAB Function1 ==
  data: x input; y output
function y = fcn(x)
%#codegen

if x
    y = 1;
else
    y = 0;
end

== matlab function SILS_201704211/SensorDataConversion/STTDataConversion/MATLAB Function2 ==
  data: x input; y output
function y = fcn(x)
%#codegen

y = [-x(2); -x(3); -x(4); x(1)];

== matlab function SILS_201704211/MATLAB Function1 ==
  data: u input; y output
function y = fcn(u)
%#codegen

v = [0; 0; -1];

u = u / norm(u);
v = v / norm(v);

costheta = u' * v;
if costheta > 1
    costheta = 1;
end
if costheta < -1
    costheta = -1;
end

y = acos(costheta) / pi * 180;

== matlab function SILS_201704211/SensorDataConversion/STTDataConversion/MATLAB Function3 ==
  data: x input; y output
function y = fcn(x)
%#codegen

y = [x(1,1); x(1,2); x(1,3); x(2,2); x(2,3); x(3,3)];
